simulink model "pid_reinforcement"  (R2023b)
settings: Solver=VariableStepAuto  StartTime=0  StopTime=40.0  RelTol=1e-3
libraries: instrumentlib x2
settings Model: Creator=pc  LastModifiedBy=pc

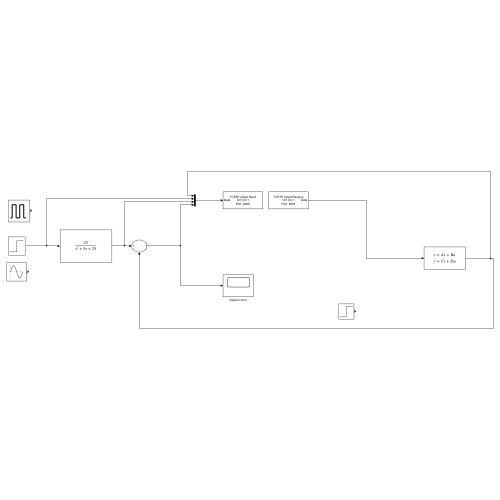
[thumbnail: Simulink's stored preview of the top-level diagram]
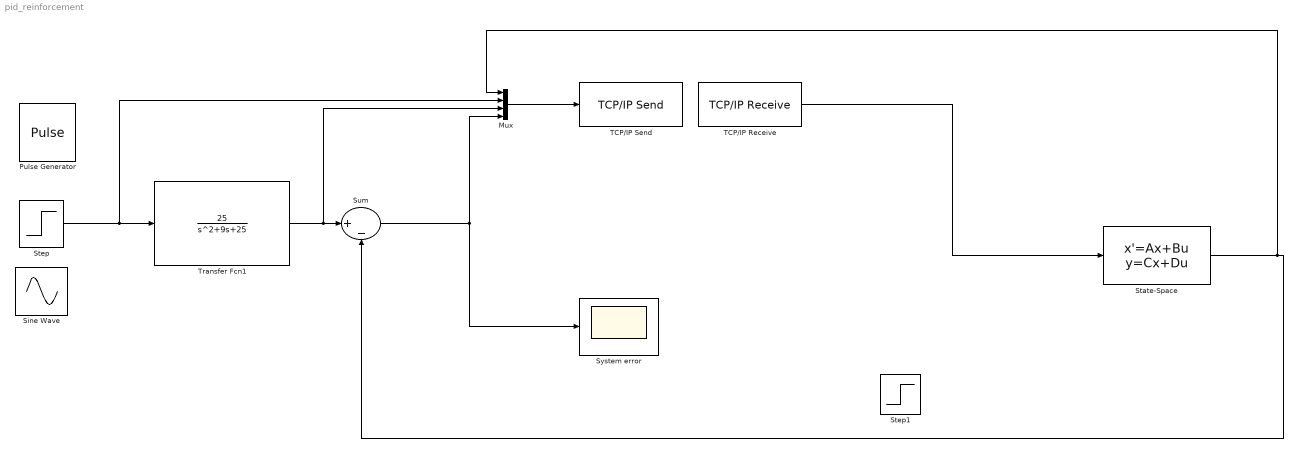
== system pid_reinforcement ==
  Mux : Mux
  Pulse Generator : DiscretePulseGenerator  PulseType=Time based  Amplitude=3  Period=10  PulseWidth=50
  Sine Wave : Sin  Amplitude=3  Frequency=4  SampleTime=0
  State-Space : StateSpace  A=3  C=2  D=0  InitialCondition=0  ParameterTunability=Optimized  ContinuousStateAttributes='Controlled_Object'
  Step : Step  Before=1  SampleTime=0
  Step1 : Step  Before=100  After=100  SampleTime=0
  Sum : Sum  Inputs=|+-
  System error : Scope
  TCP/IP Receive : instrumentlib/TCP//IP Receive  Host=127.0.0.1  Port=8281  DataSize=[ 1 ]  DataType=double  ASCIIFormatting=%f  Terminator=LF  CustomTerminator=10  ByteOrder=big-endian  EnableBlockingMode=on  Timeout=1000  SampleTime=0.01  SimulateUsing=Interpreted execution
  TCP/IP Send : instrumentlib/TCP//IP Send  Host=127.0.0.1  Port=8280  ByteOrder=big-endian  EnableBlockingMode=on  Timeout=1000  TransferDelay=on  SimulateUsing=Interpreted execution
  Transfer Fcn1 : TransferFcn  Numerator=[25]  Denominator=[1 9 25]  ContinuousStateAttributes='Reference_Model'
  wires:
  Sum/1 -> Mux/4, System error/1
  State-Space/1 -> Mux/1, Sum/2
  Transfer Fcn1/1 -> Mux/3, Sum/1
  Mux/1 -> TCP/IP Send/1
  TCP/IP Receive/1 -> State-Space/1
  Step/1 -> Mux/2, Transfer Fcn1/1
